simulink model "OMSim"  (Simulink 7.0)
settings: Solver=ode4  SolverMode=SingleTasking  StartTime=0.0  StopTime=5  FixedStep=0.001  MaxStep=0.001  RelTol=1e-3  AbsTol=1e-3
CloseFcn:
  | ;slview('closediagram',bdroot);
settings Model: Creator=jacobs  LastModifiedBy=lfd  ExtModeAutoUpdateStatusClock=off
settings DataIOCC: LimitDataPoints=off  SaveOutput=off  SaveTime=off
settings OptimizationCC: BlockReduction=off  BooleanDataType=off
settings DebuggingCC: SaveWithParameterizedLinksMsg=none  SignalResolutionControl=TryResolveAllWithWarning  SolverPrmCheckMsg=none  MultiTaskDSMMsg=warning  MultiTaskCondExecSysMsg=none  StrictBusMsg=None
settings HardwareCC: TargetUnknown=on
settings RTWCC: IncludeERTFirstTime=on
settings GRTTargetCC: TargetFcnLib=ansi_tfl_tmw.mat  ModelReferenceCompliant=off  MatFileLogging=off

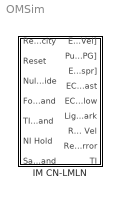
== system OMSim ==
  IM CN-LMLN : Subsystem  Orientation=left
      mask Display: disp('INTERNAL\nMONITOR')

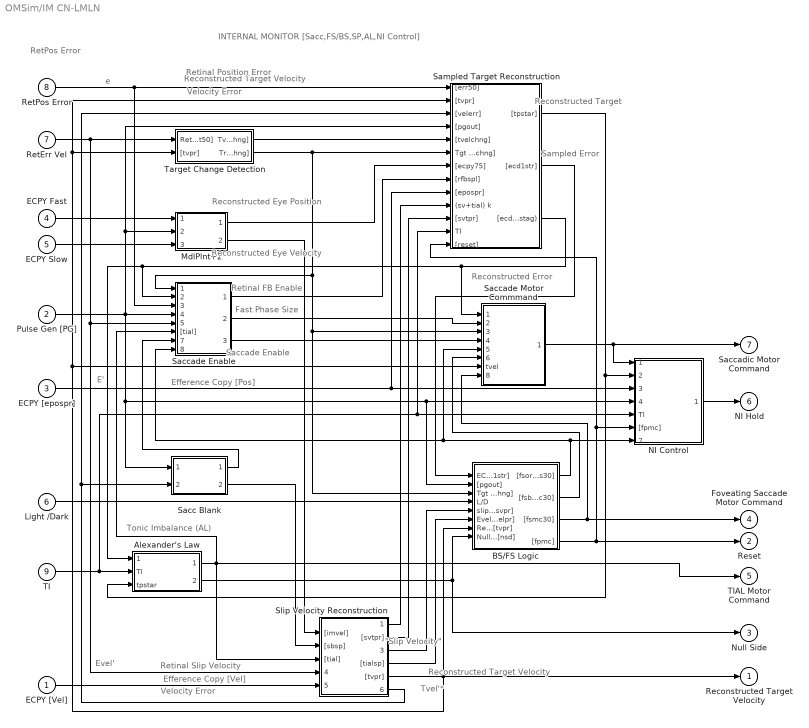
== system OMSim/IM CN-LMLN ==
  note: Velocity Error
  note: Reconstructed Target Velocity
  note: "Slip
      | Velocity"
  note: E'
  note: Efference Copy [Pos]
  note: Tvel'*
  note: Reconstructed
      | Target Velocity
  note: Efference Copy [Vel]
  note: Retinal Slip Velocity
  note: Velocity Error
  note: Evel'
  note: Fast Phase
      | Size
  note: Saccade
      | Enable
  note: Retinal FB
      | Enable
  note: Reconstructed
      | Eye Velocity
  note: Reconstructed
      | Eye Position
  note: RetPos
      | Error
  note: Retinal Position Error
  note: e
  note: Tonic Imbalance (AL)
  note: Reconstructed
      | Error
  note: Sampled
      | Error
  note: Reconstructed
      | Target
  note: INTERNAL MONITOR [Sacc,FS/BS,SP,AL,NI Control]
  ECPY [Vel] : Inport  OutDataType=sfix(16)  OutScaling=2^0
  Pulse Gen [PG] : Inport  Port=2  OutDataType=sfix(16)  OutScaling=2^0
  ECPY [epospr] : Inport  Port=3  OutDataType=sfix(16)  OutScaling=2^0
  ECPY Fast : Inport  Port=4  OutDataType=sfix(16)  OutScaling=2^0
  ECPY Slow : Inport  Port=5  OutDataType=sfix(16)  OutScaling=2^0
  Light /Dark : Inport  Port=6  OutDataType=sfix(16)  OutScaling=2^0
  RetErr Vel : Inport  Port=7  OutDataType=sfix(16)  OutScaling=2^0
  RetPos Error : Inport  Port=8  OutDataType=sfix(16)  OutScaling=2^0
  TI : Inport  Port=9  OutDataType=sfix(16)  OutScaling=2^0
  Alexander's Law : Subsystem
      mask Display: disp('Alexander''s\nLaw')
  BS/FS Logic : Subsystem
      mask Display: disp('Braking/Foveating\nSaccade\nLogic')
  MdlPlnt+2 : Subsystem
      mask Display: disp('Model\nPlant+')
  NI Control : Subsystem
      mask Display: disp('NI\nControl')
  Sacc Blank : Subsystem
      mask Display: disp('Saccade\n& Drift\nBlanking')
  Saccade Enable : Subsystem
      mask Display: disp('Saccade\nEnable')
  Saccade Motor Commmand : Subsystem
      mask Display: disp('Saccade\nMotor\nCommand')
  Sampled Target Reconstruction : Subsystem
      mask Display: disp('Sampled\nTarget & Error\nReconstruction')
  Slip Velocity Reconstruction : Subsystem
      mask Display: disp('Target &\nSlip Velocity\nReconstruction')
  Target Change Detection : Subsystem
      mask Display: disp('Target Change\nDetection')
  Reconstructed Target Velocity : Outport  OutDataType=sfix(16)  OutScaling=2^0  InitialOutput=0
  Reset : Outport  Port=2  OutDataType=sfix(16)  OutScaling=2^0  InitialOutput=0
  Null Side : Outport  Port=3  OutDataType=sfix(16)  OutScaling=2^0  InitialOutput=0
  Foveating Saccade Motor Command : Outport  Port=4  OutDataType=sfix(16)  OutScaling=2^0  InitialOutput=0
  TIAL Motor Command : Outport  Port=5  OutDataType=sfix(16)  OutScaling=2^0  InitialOutput=0
  NI Hold : Outport  Port=6  OutDataType=sfix(16)  OutScaling=2^0  InitialOutput=0
  Saccadic Motor Command : Outport  Port=7  OutDataType=sfix(16)  OutScaling=2^0  InitialOutput=0
  wires:
  Saccade Enable/2(FPh Size [fphsz]) -> Saccade Motor Commmand/2("[fphsz]")
  BS/FS Logic/4("[fpmc]") -> NI Control/6("[fpmc]"), Sampled Target Reconstruction/13("[reset]"), Reset/1
  ECPY Slow/1 -> MdlPlnt+2/3("[epossps]")
  Alexander's Law/2(Null Side [nsd]) -> Null Side/1, BS/FS Logic/8(Null Side [nsd])
  BS/FS Logic/2("[fsbsmc30]") -> Saccade Motor Commmand/6("[fsbcmc30]")
  Saccade Enable/3("[sacenab]") -> Saccade Motor Commmand/4("[sacenab]")
  Sampled Target Reconstruction/3("[ecdstrdz] (excl nystag)") -> Saccade Motor Commmand/1("[ecdstrdz]"), Alexander's Law/1(reconstructed  error), Saccade Enable/2("[ecdstrdz]")
  Sacc Blank/1(SacBlnk [sbsac]) -> Saccade Enable/7("[sbsac]")
  Slip Velocity Reconstruction/4("[tialsp]") -> BS/FS Logic/6(Evel' [evelpr])
  Slip Velocity Reconstruction/3("'slip vel\" [svpr]") -> BS/FS Logic/5(slip vel [svpr])
  Light /Dark/1 -> BS/FS Logic/4(L/D)
  Sampled Target Reconstruction/2("[ecd1str]") -> BS/FS Logic/1(ECD1* [ecd1str])
  ECPY [Vel]/1 -> Slip Velocity Reconstruction/5("[evelpr]")
  Sacc Blank/2(SP S/H [sbsp]) -> Slip Velocity Reconstruction/2("[sbsp]")
  MdlPlnt+2/2("[imvel]") -> Slip Velocity Reconstruction/1("[imvel]")
  BS/FS Logic/3("[fsmc30]") -> Foveating Saccade Motor Command/1, Saccade Motor Commmand/8(fsmc30)
  BS/FS Logic/1("[fsorbs30]") -> NI Control/7("[fsorbs30]"), Saccade Motor Commmand/5("[fsorbs30]"), Saccade Enable/8("[fsorbs30]")
  Slip Velocity Reconstruction/5("[tvpr]") -> BS/FS Logic/7(Recon Tgt Vel [tvpr]), Saccade Motor Commmand/7(tvel), Sampled Target Reconstruction/2("[tvpr]"), Target Change Detection/2("[tvpr]"), Reconstructed Target Velocity/1
  Saccade Enable/1("[rfbspl]") -> Sampled Target Reconstruction/8("[rfbspl]")
  MdlPlnt+2/1("[ecpy80]") -> Sampled Target Reconstruction/7("[ecpy75]")
  RetPos Error/1 -> Sampled Target Reconstruction/1("[err50]"), Saccade Enable/3("[err50]")
  Sampled Target Reconstruction/1("[tpstar]") -> Alexander's Law/3(tpstar), NI Control/2(T'* [tpstar])
  Target Change Detection/1(Tvel Chng [tvelchng]) -> Sampled Target Reconstruction/5("[tvelchng]")
  Slip Velocity Reconstruction/6("[velerr]") -> Sacc Blank/2(RetVelErr [velerr]), Sampled Target Reconstruction/3("[velerr]")
  Slip Velocity Reconstruction/2("[svtpr]") -> Sampled Target Reconstruction/11("[svtpr]")
  Slip Velocity Reconstruction/1(Vel->Pos) -> Sampled Target Reconstruction/10((sv+tial) k)
  RetErr Vel/1 -> Slip Velocity Reconstruction/4("[edot50]"), Saccade Enable/5("[edot50]"), Target Change Detection/1(RetErr Vel [edot50])
  Target Change Detection/2(Trgt Chng [tchng]) -> Saccade Enable/1(Tgt ch Det [tchng]), Saccade Motor Commmand/3(Tgt ch Det [tchng]), BS/FS Logic/3(Tgt ch Det [tchng]), Sampled Target Reconstruction/6(Tgt ch Det [tchng])
  Saccade Motor Commmand/1("[posmc]") -> Saccadic Motor Command/1, NI Control/1("[posmc]")
  Alexander's Law/1(TIAL [tial]) -> TIAL Motor Command/1, Saccade Enable/6("[tial]"), Slip Velocity Reconstruction/3("[tial]")
  ECPY Fast/1 -> MdlPlnt+2/1("[eposspf]")
  Pulse Gen [PG]/1 -> MdlPlnt+2/2("[pgout]"), Sampled Target Reconstruction/4("[pgout]"), Saccade Enable/4("[pgout]"), BS/FS Logic/2("[pgout]"), NI Control/4(PG [pgout]), Sacc Blank/1(PG [pgout])
  TI/1 -> Alexander's Law/2(TI), Sampled Target Reconstruction/12(TI), NI Control/5(TI)
  ECPY [epospr]/1 -> Sampled Target Reconstruction/9("[epospr]"), NI Control/3("[epospr]")
  NI Control/1(Hold [nihold]) -> NI Hold/1

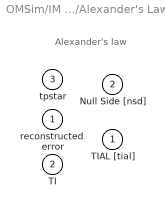
== system OMSim/IM CN-LMLN/Alexander's Law ==
  note: Alexander's law
  reconstructed  error : Inport  OutDataType=sfix(16)  OutScaling=2^0
  TI : Inport  Port=2  OutDataType=sfix(16)  OutScaling=2^0
  tpstar : Inport  Port=3  OutDataType=sfix(16)  OutScaling=2^0
  TIAL [tial] : Outport  OutDataType=sfix(16)  OutScaling=2^0  InitialOutput=0
  Null Side [nsd] : Outport  Port=2  OutDataType=sfix(16)  OutScaling=2^0  InitialOutput=0

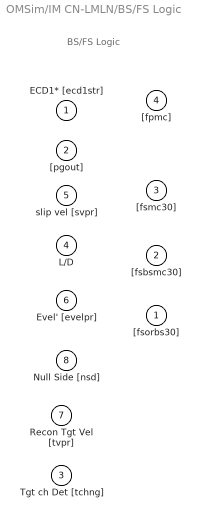
== system OMSim/IM CN-LMLN/BS/FS Logic ==
  note: BS/FS Logic
  ECD1* [ecd1str] : Inport  OutDataType=sfix(16)  OutScaling=2^0
  "[pgout]" : Inport  Port=2  OutDataType=sfix(16)  OutScaling=2^0
  Tgt ch Det [tchng] : Inport  Port=3  OutDataType=sfix(16)  OutScaling=2^0
  L/D : Inport  Port=4  OutDataType=sfix(16)  OutScaling=2^0
  slip vel [svpr] : Inport  Port=5  OutDataType=sfix(16)  OutScaling=2^0
  Evel' [evelpr] : Inport  Port=6  OutDataType=sfix(16)  OutScaling=2^0
  Recon Tgt Vel [tvpr] : Inport  Port=7  OutDataType=sfix(16)  OutScaling=2^0
  Null Side [nsd] : Inport  Port=8  OutDataType=sfix(16)  OutScaling=2^0
  "[fsorbs30]" : Outport  OutDataType=sfix(16)  OutScaling=2^0  InitialOutput=0
  "[fsbsmc30]" : Outport  Port=2  OutDataType=sfix(16)  OutScaling=2^0  InitialOutput=0
  "[fsmc30]" : Outport  Port=3  OutDataType=sfix(16)  OutScaling=2^0  InitialOutput=0
  "[fpmc]" : Outport  Port=4  OutDataType=sfix(16)  OutScaling=2^0  InitialOutput=0

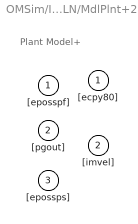
== system OMSim/IM CN-LMLN/MdlPlnt+2 ==
  note: Plant Model+
  "[eposspf]" : Inport  OutDataType=sfix(16)  OutScaling=2^0
  "[pgout]" : Inport  Port=2  OutDataType=sfix(16)  OutScaling=2^0
  "[epossps]" : Inport  Port=3  OutDataType=sfix(16)  OutScaling=2^0
  "[ecpy80]" : Outport  OutDataType=sfix(16)  OutScaling=2^0  InitialOutput=0
  "[imvel]" : Outport  Port=2  OutDataType=sfix(16)  OutScaling=2^0  InitialOutput=0

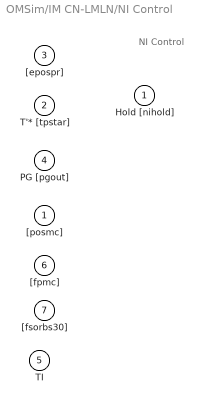
== system OMSim/IM CN-LMLN/NI Control ==
  note: NI Control
  "[posmc]" : Inport  OutDataType=sfix(16)  OutScaling=2^0
  T'* [tpstar] : Inport  Port=2  OutDataType=sfix(16)  OutScaling=2^0
  "[epospr]" : Inport  Port=3  OutDataType=sfix(16)  OutScaling=2^0
  PG [pgout] : Inport  Port=4  OutDataType=sfix(16)  OutScaling=2^0
  TI : Inport  Port=5  OutDataType=sfix(16)  OutScaling=2^0
  "[fpmc]" : Inport  Port=6  OutDataType=sfix(16)  OutScaling=2^0
  "[fsorbs30]" : Inport  Port=7  OutDataType=sfix(16)  OutScaling=2^0
  Hold [nihold] : Outport  OutDataType=sfix(16)  OutScaling=2^0  InitialOutput=0

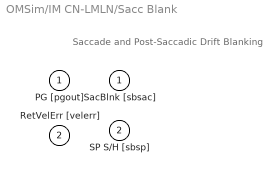
== system OMSim/IM CN-LMLN/Sacc Blank ==
  note: Saccade and Post-Saccadic Drift Blanking
  PG [pgout] : Inport  OutDataType=sfix(16)  OutScaling=2^0
  RetVelErr [velerr] : Inport  Port=2  OutDataType=sfix(16)  OutScaling=2^0
  SacBlnk [sbsac] : Outport  OutDataType=sfix(16)  OutScaling=2^0  InitialOutput=0
  SP S/H [sbsp] : Outport  Port=2  OutDataType=sfix(16)  OutScaling=2^0  InitialOutput=0

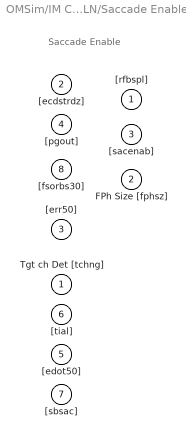
== system OMSim/IM CN-LMLN/Saccade Enable ==
  note: Saccade Enable
  Tgt ch Det [tchng] : Inport  OutDataType=sfix(16)  OutScaling=2^0
  "[ecdstrdz]" : Inport  Port=2  OutDataType=sfix(16)  OutScaling=2^0
  "[err50]" : Inport  Port=3  OutDataType=sfix(16)  OutScaling=2^0
  "[pgout]" : Inport  Port=4  OutDataType=sfix(16)  OutScaling=2^0
  "[edot50]" : Inport  Port=5  OutDataType=sfix(16)  OutScaling=2^0
  "[tial]" : Inport  Port=6  OutDataType=sfix(16)  OutScaling=2^0
  "[sbsac]" : Inport  Port=7  OutDataType=sfix(16)  OutScaling=2^0
  "[fsorbs30]" : Inport  Port=8  OutDataType=sfix(16)  OutScaling=2^0
  "[rfbspl]" : Outport  OutDataType=sfix(16)  OutScaling=2^0  InitialOutput=0
  FPh Size [fphsz] : Outport  Port=2  OutDataType=sfix(16)  OutScaling=2^0  InitialOutput=0
  "[sacenab]" : Outport  Port=3  OutDataType=sfix(16)  OutScaling=2^0  InitialOutput=0

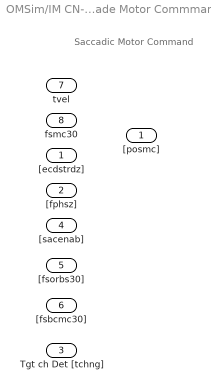
== system OMSim/IM CN-LMLN/Saccade Motor Commmand ==
  note: Saccadic Motor Command
  "[ecdstrdz]" : Inport  OutDataType=sfix(16)  OutScaling=2^0
  "[fphsz]" : Inport  Port=2  OutDataType=sfix(16)  OutScaling=2^0
  Tgt ch Det [tchng] : Inport  Port=3  OutDataType=sfix(16)  OutScaling=2^0
  "[sacenab]" : Inport  Port=4  OutDataType=sfix(16)  OutScaling=2^0
  "[fsorbs30]" : Inport  Port=5  OutDataType=sfix(16)  OutScaling=2^0
  "[fsbcmc30]" : Inport  Port=6  OutDataType=sfix(16)  OutScaling=2^0
  tvel : Inport  Port=7  OutDataType=sfix(16)  OutScaling=2^0
  fsmc30 : Inport  Port=8  OutDataType=sfix(16)  OutScaling=2^0
  "[posmc]" : Outport  OutDataType=sfix(16)  OutScaling=2^0  InitialOutput=0

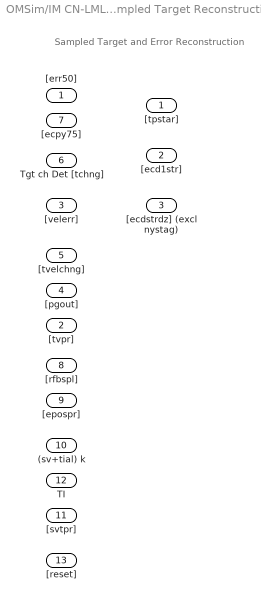
== system OMSim/IM CN-LMLN/Sampled Target Reconstruction ==
  note: Sampled Target and Error Reconstruction
  "[err50]" : Inport  OutDataType=sfix(16)  OutScaling=2^0
  "[tvpr]" : Inport  Port=2  OutDataType=sfix(16)  OutScaling=2^0
  "[velerr]" : Inport  Port=3  OutDataType=sfix(16)  OutScaling=2^0
  "[pgout]" : Inport  Port=4  OutDataType=sfix(16)  OutScaling=2^0
  "[tvelchng]" : Inport  Port=5  OutDataType=sfix(16)  OutScaling=2^0
  Tgt ch Det [tchng] : Inport  Port=6  OutDataType=sfix(16)  OutScaling=2^0
  "[ecpy75]" : Inport  Port=7  OutDataType=sfix(16)  OutScaling=2^0
  "[rfbspl]" : Inport  Port=8  OutDataType=sfix(16)  OutScaling=2^0
  "[epospr]" : Inport  Port=9  OutDataType=sfix(16)  OutScaling=2^0
  (sv+tial) k : Inport  Port=10  OutDataType=sfix(16)  OutScaling=2^0
  "[svtpr]" : Inport  Port=11  OutDataType=sfix(16)  OutScaling=2^0
  TI : Inport  Port=12  OutDataType=sfix(16)  OutScaling=2^0
  "[reset]" : Inport  Port=13  OutDataType=sfix(16)  OutScaling=2^0
  "[tpstar]" : Outport  OutDataType=sfix(16)  OutScaling=2^0  InitialOutput=0
  "[ecd1str]" : Outport  Port=2  OutDataType=sfix(16)  OutScaling=2^0  InitialOutput=0
  "[ecdstrdz] (excl nystag)" : Outport  Port=3  OutDataType=sfix(16)  OutScaling=2^0  InitialOutput=0

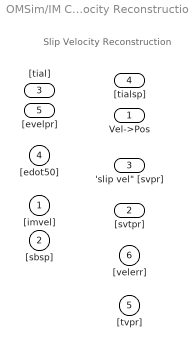
== system OMSim/IM CN-LMLN/Slip Velocity Reconstruction ==
  note: Slip Velocity Reconstruction
  "[imvel]" : Inport  OutDataType=sfix(16)  OutScaling=2^0
  "[sbsp]" : Inport  Port=2  OutDataType=sfix(16)  OutScaling=2^0
  "[tial]" : Inport  Port=3  OutDataType=sfix(16)  OutScaling=2^0
  "[edot50]" : Inport  Port=4  OutDataType=sfix(16)  OutScaling=2^0
  "[evelpr]" : Inport  Port=5  OutDataType=sfix(16)  OutScaling=2^0
  Vel->Pos : Outport  OutDataType=sfix(16)  OutScaling=2^0  InitialOutput=0
  "[svtpr]" : Outport  Port=2  OutDataType=sfix(16)  OutScaling=2^0  InitialOutput=0
  "'slip vel\" [svpr]" : Outport  Port=3  OutDataType=sfix(16)  OutScaling=2^0  InitialOutput=0
  "[tialsp]" : Outport  Port=4  OutDataType=sfix(16)  OutScaling=2^0  InitialOutput=0
  "[tvpr]" : Outport  Port=5  OutDataType=sfix(16)  OutScaling=2^0  InitialOutput=0
  "[velerr]" : Outport  Port=6  OutDataType=sfix(16)  OutScaling=2^0  InitialOutput=0

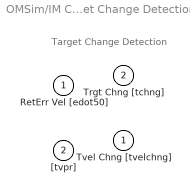
== system OMSim/IM CN-LMLN/Target Change Detection ==
  note: Target Change Detection
  RetErr Vel [edot50] : Inport  OutDataType=sfix(16)  OutScaling=2^0
  "[tvpr]" : Inport  Port=2  OutDataType=sfix(16)  OutScaling=2^0
  Tvel Chng [tvelchng] : Outport  OutDataType=sfix(16)  OutScaling=2^0  InitialOutput=0
  Trgt Chng [tchng] : Outport  Port=2  OutDataType=sfix(16)  OutScaling=2^0  InitialOutput=0
